simulink model "Wind_Harness"  (R2025b)
settings: Solver=VariableStepAuto  StartTime=0.0  StopTime=5  FixedStep=5e-5  RelTol=1e-3
PostLoadFcn:
  | WindFarmParam;
values from neighbouring files (symbols this model uses):
  base = struct    [WindFarmParam.m]
  pmsm = struct    [WindFarmParam.m]
  Ts = 5E-5    (= 5e-05)    [BESSGFLParam.m]    (also in BESSGFMParam.m; WindFarmParam.m)
  windController = struct    [WindFarmParam.m]
  windSystem = struct    [WindFarmParam.m]
  windTurbine = saveVarsMat.windTurbine    [WindFarmParam.m]
undefined symbols (not defined in the file or in its folder): DiscIntNeverNeededParam, Inertia
libraries: nesl_utility x34, fl_lib x18, ee_lib x18, eeTransforms x6, eeGeneralControl x5, simulink x4, eePwmGenerator x2, eeSinusoidalMeasurementV2 x1, eePmsmCurrentController x1, custom_lib x1
(part 2 of 2)

== system Wind_Harness/Wind Plant/Detailed/Wind Turbine and Converters/Wind Plant/Back-to-Back Converters ==
  Chopper : Inport
  SM_ref : Inport  Port=2
  Grid_ref : Inport  Port=3
  Average : Subsystem  VariantControl=Average
  Switching : Subsystem  VariantControl=Switching
  In : PMIOPort  Side=Left
  ~ : PMIOPort  Port=2  Side=Right
  Vdc : Outport

== system Wind_Harness/Wind Plant/Detailed/Wind Turbine and Converters/Wind Controller/Machine Converter Control/Measurements ==
  iabc_sens : Inport
  w_sens : Inport  Port=2
  th_sens : Inport  Port=3
  Vdc_sens : Inport  Port=4
  2*pi : Constant  Value=2*pi  SampleTime=-1
  Math Function : Math  Operator=mod  SignedPower=on
  pole pairs : Gain  Gain=p
  "pole pairs " : Gain  Gain=p
  we : Outport  VectorParamsAs1DForOutWhenUnconnected=off
  iabc : Outport  Port=2  VectorParamsAs1DForOutWhenUnconnected=off
  theta : Outport  Port=3  VectorParamsAs1DForOutWhenUnconnected=off
  Vdc : Outport  Port=4  VectorParamsAs1DForOutWhenUnconnected=off
  wires:
  Math Function/1 -> theta/1
  Vdc_sens/1 -> Vdc/1
  "pole pairs "/1 -> Math Function/1
  th_sens/1 -> "pole pairs "/1
  2*pi/1 -> Math Function/2
  pole pairs/1 -> we/1
  iabc_sens/1 -> iabc/1
  w_sens/1 -> pole pairs/1

== system Wind_Harness/Wind Plant/Detailed/Wind Turbine and Converters/Wind Controller/Machine Converter Control/Power Controller ==
  windSpeed : Inport
  Derating Control : Subsystem
  Greater than : simulink/Logic and Bit Operations/Compare To Constant  relop=>  const=12  OutDataTypeStr=boolean
  Less than or equal to : simulink/Logic and Bit Operations/Compare To Constant  relop=<=  const=12  OutDataTypeStr=boolean
  Limiter Function Power Demand : Subsystem
  MPPT Control : Subsystem
  activePowerDemand : Outport
  wires:
  Limiter Function Power Demand/1(activePowerDemand) -> activePowerDemand/1
  Derating Control/1(activePowerDemand) -> Limiter Function Power Demand/2(activePowerDemandDerating)
  MPPT Control/1(activePowerDemand) -> Limiter Function Power Demand/1(activePowerDemandMPPT)
  Greater than/1 -> Derating Control/Enable
  Less than or equal to/1 -> MPPT Control/Enable
  windSpeed/1 -> MPPT Control/1(windSpeed), Less than or equal to/1, Greater than/1

== system Wind_Harness/Wind Plant/Detailed/Wind Turbine and Converters/Wind Controller/Machine Converter Control/Subsystem ==
  note: LVRT Crowbar Control
  Vdc : Inport
  LVRT : Inport  Port=2
  Abs : Abs  SaturateOnIntegerOverflow=off
  Constant1 : Constant  Value=Vdc
  Product : Product
  Relay : Relay  OnSwitchValue=0.01001*Vdc  OffSwitchValue=0.01*Vdc
  Sum : Sum  Inputs=|+-
  Unit Delay1 : UnitDelay  SampleTime=-1  HasFrameUpgradeWarning=on
  Out1 : Outport
  wires:
  Relay/1 -> Out1/1
  Product/1 -> Abs/1
  LVRT/1 -> Product/2
  Unit Delay1/1 -> Sum/2
  Abs/1 -> Relay/1
  Sum/1 -> Product/1
  Vdc/1 -> Unit Delay1/1
  Constant1/1 -> Sum/1

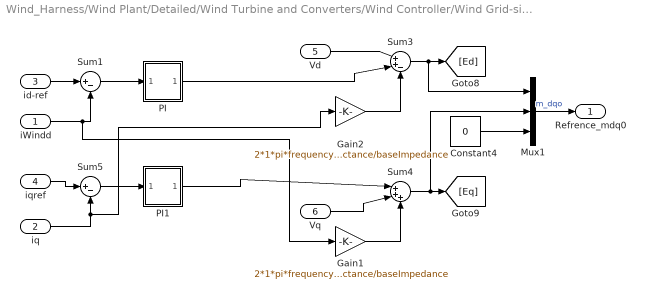
== system Wind_Harness/Wind Plant/Detailed/Wind Turbine and Converters/Wind Controller/Wind Grid-side Converter Controller/Current_controller ==
  iWindd : Inport
  iq : Inport  Port=2
  id-ref : Inport  Port=3
  iqref : Inport  Port=4
  Vd : Inport  Port=5
  Vq : Inport  Port=6
  Constant4 : Constant  Value=0
  Gain1 : Gain  Gain=2*1*pi*frequency*inductance/baseImpedance
  Gain2 : Gain  Gain=2*1*pi*frequency*inductance/baseImpedance
  Mux1 : Mux  Inputs=3
  PI : Subsystem
  PI1 : Subsystem
  Sum1 : Sum  Inputs=|+-
  Sum3 : Sum  Inputs=|++-
  Sum4 : Sum  Inputs=|+++
  Sum5 : Sum  Inputs=|+-
  Refrence_mdq0 : Outport
  wires:
  Mux1/1 -> Refrence_mdq0/1  "m_dqo"
  Sum4/1 -> [Eq], Mux1/2
  PI1/1(Out2) -> Sum4/1
  iqref/1 -> Sum5/1
  Sum5/1 -> PI1/1(Input)
  Constant4/1 -> Mux1/3
  Vd/1 -> Sum3/1
  Sum1/1 -> PI/1(Input)
  iq/1 -> Sum5/2, Gain2/1
  Vq/1 -> Sum4/2
  Gain1/1 -> Sum4/3
  id-ref/1 -> Sum1/1
  iWindd/1 -> Sum1/2, Gain1/1
  Gain2/1 -> Sum3/3
  Sum3/1 -> [Ed], Mux1/1
  PI/1(Out2) -> Sum3/2

== system Wind_Harness/Wind Plant/Detailed/Wind Turbine and Converters/Wind Controller/Wind Grid-side Converter Controller/DC Bus Chopper control  ==
  note: LVRT Detection
  In1 : Inport
  Constant1 : Constant
  Constant2 : Constant  Value=0
  Switch : Switch  Criteria=u2 > Threshold  Threshold=0.9  SaturateOnIntegerOverflow=off  InputSameDT=off
  Unit Delay : UnitDelay  SampleTime=-1  HasFrameUpgradeWarning=on
  Out1 : Outport
  wires:
  Unit Delay/1 -> Switch/2
  In1/1 -> Unit Delay/1
  Constant2/1 -> Switch/1
  Constant1/1 -> Switch/3
  Switch/1 -> Out1/1

== system Wind_Harness/Wind Plant/Detailed/Wind Turbine and Converters/Wind Controller/Wind Grid-side Converter Controller/DC voltage controller & current reference ==
  note: id_ref_generator
  note: iq_ref_generator
  note: Limiter
  Q_ref : Inport
  Vmag : Inport  Port=2
  Wind_Mpp_vdc : Inport  Port=3
  Wind_vdc : Inport  Port=4
  lvrt.iq : Inport  Port=5
  Constant : Constant
  Constant1 : Constant  Value=iMaxPU
  Current limits : Subsystem
  Subsystem : Subsystem
  Subsystem1 : Subsystem
  Switch : Switch  Criteria=u2 > Threshold  SaturateOnIntegerOverflow=off  InputSameDT=off
  Unit Delay1 : UnitDelay  SampleTime=Ts  HasFrameUpgradeWarning=on
  Unit Delay3 : UnitDelay  SampleTime=Ts  HasFrameUpgradeWarning=on
  id_ref : Outport
  iq_ref : Outport  Port=2
  wires:
  Constant/1 -> Switch/3
  Switch/1 -> Subsystem/1(V_mag)
  Vmag/1 -> Switch/2, Switch/1
  lvrt.iq/1 -> Subsystem/3(lvrt.iq)
  Current limits/1(iubq) -> Subsystem/2(iq_ub)
  Wind_vdc/1 -> Subsystem1/2(Wind_vdc)
  Wind_Mpp_vdc/1 -> Subsystem1/1(Wind_Mpp_vdc)
  Q_ref/1 -> Subsystem/4(Q_ref)
  Unit Delay3/1 -> Current limits/3(idref)
  Subsystem1/1(Out1) -> Unit Delay3/1, id_ref/1
  Unit Delay1/1 -> Current limits/2(iqref)
  Constant1/1 -> Current limits/1(Imax)
  Subsystem/1(Out1) -> iq_ref/1, Unit Delay1/1
  Current limits/2(iubd) -> Subsystem1/3(id_ub)

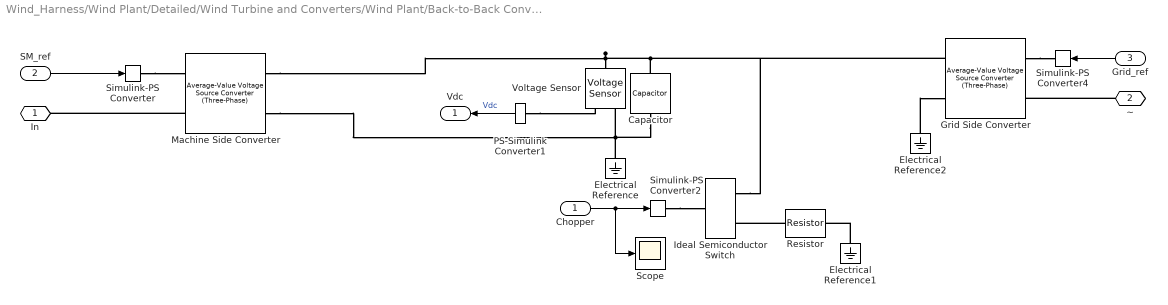
== system Wind_Harness/Wind Plant/Detailed/Wind Turbine and Converters/Wind Plant/Back-to-Back Converters/Average ==
  Chopper : Inport
  SM_ref : Inport  Port=2
  Grid_ref : Inport  Port=3
  Capacitor : fl_lib/Electrical/Electrical Elements/Capacitor  c=capDC F  r=1e-1 Ohm  g=0 1/Ohm  i_specify=off  i_priority=None  i=0 A  i_nominal_specify=off  i_nominal_value=1  i_nominal_unit=A  v_specify=off  v_priority=None  v=0 V  v_nominal_specify=off  v_nominal_value=1  v_nominal_unit=V  vc_specify=on  vc_priority=High  vc=Vdc V  vc_nominal_specify=off  vc_nominal_value=1  vc_nominal_unit=V
  Electrical Reference : fl_lib/Electrical/Electrical Elements/Electrical Reference
  Electrical Reference1 : fl_lib/Electrical/Electrical Elements/Electrical Reference
  Electrical Reference2 : fl_lib/Electrical/Electrical Elements/Electrical Reference
  Grid Side Converter : ee_lib/Semiconductors & Converters/Converters/Average-Value Voltage Source Converter (Three-Phase)  port_option=ee.enum.threePhasePort.composite  frequency_option=ee.enum.converters.frequency.variable  input_option=ee.enum.converters.inputOption.ModWave  FRated=60 Hz  losses_parameterization=ee.enum.converters.losses.fixed  Pfixed=1 W  ks=0.01  kc1=1.7 V  kc2=0.01 Ohm  Ploss_vect=[100, 800, 1870, 3250, 4900] W  Irms_vect=[10, 100, 200, 300, 400] A  Vdc_nom=300 V  thermal_mass=30000 J/K  temperature_specify=off  temperature_priority=High  temperature=298.15 K  temperature_nominal_specify=off  temperature_nominal_value=1  temperature_nominal_unit=K
      settings: InternalSimscapePortConfiguration="{\"Bottom\":[],\"Left\":[{\"id\":\"ModWave\",\"label\":\"ModWave\",\"type\":\"input\"},{\"id\":\"N\",\"label\":\"~\",\"type\":\"foundation.electrical.three_phase\"}],\"Right\":[{\"id\":\"p\",\"label\":\"+\",\"type\":\"foundation.electrical.electrical\"},{\"id\":\"n\",\"label\":\"-\",\"type\":\"foundation.electrical.electrical\"}],\"Top\":[]}"
  Ideal Semiconductor Switch : ee_lib/Semiconductors & Converters/Ideal Semiconductor Switch  port_option=ee.enum.controlport.ps  Ron=0.001 Ohm  Goff=1e-6 1/Ohm  Vth=0.5 V  diode_param=ee.enum.converters.protectiondiode.none  diode_Vf=0.8 V  diode_Ron=0.001 Ohm  diode_Goff=1e-5 1/Ohm  diode_C=50e-9 F  diode_iRM=-235 A  diode_iF=300 A  diode_idot=-50 A/us  diode_trr_param=ee.enum.converters.diodetrr.trr_factor  diode_trr_factor=3  diode_trr=15 us  diode_Qrr=1500 s*uA
  Machine Side Converter : ee_lib/Semiconductors & Converters/Converters/Average-Value Voltage Source Converter (Three-Phase)  port_option=ee.enum.threePhasePort.composite  frequency_option=ee.enum.converters.frequency.variable  input_option=ee.enum.converters.inputOption.ModWave  FRated=60 Hz  losses_parameterization=ee.enum.converters.losses.fixed  Pfixed=1 W  ks=0.01  kc1=1.7 V  kc2=0.01 Ohm  Ploss_vect=[100, 800, 1870, 3250, 4900] W  Irms_vect=[10, 100, 200, 300, 400] A  Vdc_nom=300 V  thermal_mass=30000 J/K  temperature_specify=off  temperature_priority=High  temperature=298.15 K  temperature_nominal_specify=off  temperature_nominal_value=1  temperature_nominal_unit=K
      settings: InternalSimscapePortConfiguration="{\"Bottom\":[],\"Left\":[{\"id\":\"ModWave\",\"label\":\"ModWave\",\"type\":\"input\"},{\"id\":\"N\",\"label\":\"~\",\"type\":\"foundation.electrical.three_phase\"}],\"Right\":[{\"id\":\"p\",\"label\":\"+\",\"type\":\"foundation.electrical.electrical\"},{\"id\":\"n\",\"label\":\"-\",\"type\":\"foundation.electrical.electrical\"}],\"Top\":[]}"
  PS-Simulink Converter1 : nesl_utility/PS-Simulink Converter  PhysicalDomain=network_engine_domain  SubClassName=ps_output  LeftPortType=input  RightPortType=output  PseudoPeriodic=off  Frequencies=[]  VectorFormat=1-D array  Unit=V  AffineConversion=off
  Resistor : fl_lib/Electrical/Electrical Elements/Resistor  R=16 Ohm  i_specify=off  i_priority=None  i=0 A  i_nominal_specify=off  i_nominal_value=1  i_nominal_unit=A  v_specify=off  v_priority=None  v=0 V  v_nominal_specify=off  v_nominal_value=1  v_nominal_unit=V
  Scope : Scope
      settings: ActiveDisplayYMinimum=-0.125  ActiveDisplayYMaximum=1.125  DataLoggingVariableName=ScopeData11
  Simulink-PS Converter : nesl_utility/Simulink-PS Converter  PhysicalDomain=network_engine_domain  SubClassName=ps_input  LeftPortType=input  RightPortType=output  PseudoPeriodic=off  Frequencies=[]  NoiseDistribution=none  NoiseParameters=[]  Unit=1  AffineConversion=off  FilteringAndDerivatives=provide  SimscapeFilterOrder=1  InputFilterTimeConstant=0.001  UdotUserProvided=0
  Simulink-PS Converter2 : nesl_utility/Simulink-PS Converter  PhysicalDomain=network_engine_domain  SubClassName=ps_input  LeftPortType=input  RightPortType=output  PseudoPeriodic=off  Frequencies=[]  NoiseDistribution=none  NoiseParameters=[]  Unit=1  AffineConversion=off  FilteringAndDerivatives=provide  SimscapeFilterOrder=1  InputFilterTimeConstant=0.001  UdotUserProvided=0
  Simulink-PS Converter4 : nesl_utility/Simulink-PS Converter  PhysicalDomain=network_engine_domain  SubClassName=ps_input  LeftPortType=input  RightPortType=output  PseudoPeriodic=off  Frequencies=[]  NoiseDistribution=none  NoiseParameters=[]  Unit=1  AffineConversion=off  FilteringAndDerivatives=provide  SimscapeFilterOrder=1  InputFilterTimeConstant=0.001  UdotUserProvided=0
  Voltage Sensor : fl_lib/Electrical/Electrical Sensors/Voltage Sensor
  In : PMIOPort  Side=Left
  ~ : PMIOPort  Port=2  Side=Right
  Vdc : Outport
  wires:
  SM_ref/1 -> Simulink-PS Converter/1
  PS-Simulink Converter1/1 -> Vdc/1  "Vdc"
  Chopper/1 -> Simulink-PS Converter2/1, Scope/1
  Grid_ref/1 -> Simulink-PS Converter4/1
  connections:
  Simulink-PS Converter/RConn1 -- Machine Side Converter/LConn1
  Machine Side Converter/LConn2 -- In/RConn1
  Simulink-PS Converter2/RConn1 -- Ideal Semiconductor Switch/LConn1
  Electrical Reference1/LConn1 -- Resistor/RConn1
  Grid Side Converter/LConn1 -- Simulink-PS Converter4/RConn1
  Resistor/LConn1 -- Ideal Semiconductor Switch/RConn2
  ~/RConn1 -- Grid Side Converter/LConn2
  PS-Simulink Converter1/LConn1 -- Voltage Sensor/RConn1
  Electrical Reference2/LConn1 -- Grid Side Converter/RConn2
  Voltage Sensor/LConn1 -- Machine Side Converter/RConn1 -- Ideal Semiconductor Switch/RConn1 -- Grid Side Converter/RConn1 -- Capacitor/LConn1
  Capacitor/RConn1 -- Voltage Sensor/RConn2 -- Machine Side Converter/RConn2 -- Electrical Reference/LConn1

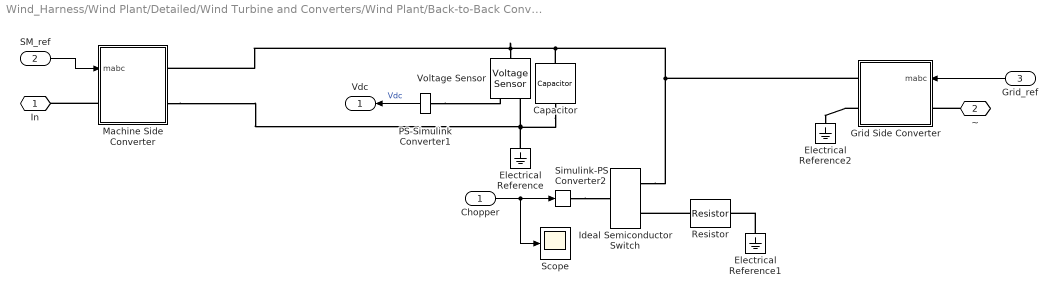
== system Wind_Harness/Wind Plant/Detailed/Wind Turbine and Converters/Wind Plant/Back-to-Back Converters/Switching ==
  Chopper : Inport
  SM_ref : Inport  Port=2
  Grid_ref : Inport  Port=3
  Capacitor : fl_lib/Electrical/Electrical Elements/Capacitor  c=capacitance F  r=1e-1 Ohm  g=0 1/Ohm  i_specify=off  i_priority=None  i=0 A  i_nominal_specify=off  i_nominal_value=1  i_nominal_unit=A  v_specify=off  v_priority=None  v=0 V  v_nominal_specify=off  v_nominal_value=1  v_nominal_unit=V  vc_specify=on  vc_priority=High  vc=baseVoltageDC V  vc_nominal_specify=off  vc_nominal_value=1  vc_nominal_unit=V
  Electrical Reference : fl_lib/Electrical/Electrical Elements/Electrical Reference
  Electrical Reference1 : fl_lib/Electrical/Electrical Elements/Electrical Reference
  Electrical Reference2 : fl_lib/Electrical/Electrical Elements/Electrical Reference
  Grid Side Converter : Subsystem
      settings: PortSchema="{\"entries\":[{\"content\":{\"sides\":[{\"content\":{\"connectorIds\":[\"LConn1\",\"LConn2\"]},\"type\":\"ConnectorPlacement.EquallySpacedRectSide\",\"uuid\":\"e32be008-cebd-46aa-ba62-c5c92b9b23e3\"},{\"content\":{\"connectorIds\":[\"In1\",\"RConn1\"],\"side\":\"RIGHT\"},\"type\":\"ConnectorPlacement.EquallySpacedRectSide\",\"uuid\":\"c483e451-04b5-4212-bdd1-c589ba5bea78\"},{\"content\":{\"side\":\"TOP\"},\"type\":\"ConnectorPlacement.EquallySpacedRectSide\",\"uuid\":\"824c135c-7e5f-4da0-a7de-e626b4bfa50d\"}]},\"type\":\"ConnectorPlacement.EquallySpacedConnector\",\"uuid\":\"5f81c72d-92ab-4525-91a6-193f769a7c86\"}],\"packageUris\":[\"http://schema.mathworks.com/mf0/Connector/R2020b\"],\"version\":\"1.0\"}"
  Ideal Semiconductor Switch : ee_lib/Semiconductors & Converters/Ideal Semiconductor Switch  port_option=ee.enum.controlport.ps  Ron=0.001 Ohm  Goff=1e-6 1/Ohm  Vth=0.5 V  diode_param=ee.enum.converters.protectiondiode.none  diode_Vf=0.8 V  diode_Ron=0.001 Ohm  diode_Goff=1e-5 1/Ohm  diode_C=50e-9 F  diode_iRM=-235 A  diode_iF=300 A  diode_idot=-50 A/us  diode_trr_param=ee.enum.converters.diodetrr.trr_factor  diode_trr_factor=3  diode_trr=15 us  diode_Qrr=1500 s*uA
  Machine Side Converter : Subsystem
      settings: PortSchema="{\"entries\":[{\"content\":{\"sides\":[{\"content\":{\"connectorIds\":[\"LConn1\",\"LConn2\"]},\"type\":\"ConnectorPlacement.EquallySpacedRectSide\",\"uuid\":\"e32be008-cebd-46aa-ba62-c5c92b9b23e3\"},{\"content\":{\"connectorIds\":[\"In1\",\"RConn1\"],\"side\":\"RIGHT\"},\"type\":\"ConnectorPlacement.EquallySpacedRectSide\",\"uuid\":\"c483e451-04b5-4212-bdd1-c589ba5bea78\"},{\"content\":{\"side\":\"TOP\"},\"type\":\"ConnectorPlacement.EquallySpacedRectSide\",\"uuid\":\"824c135c-7e5f-4da0-a7de-e626b4bfa50d\"}]},\"type\":\"ConnectorPlacement.EquallySpacedConnector\",\"uuid\":\"5f81c72d-92ab-4525-91a6-193f769a7c86\"}],\"packageUris\":[\"http://schema.mathworks.com/mf0/Connector/R2020b\"],\"version\":\"1.0\"}"
  PS-Simulink Converter1 : nesl_utility/PS-Simulink Converter  PhysicalDomain=network_engine_domain  SubClassName=ps_output  LeftPortType=input  RightPortType=output  PseudoPeriodic=off  Frequencies=[]  VectorFormat=1-D array  Unit=V  AffineConversion=off
  Resistor : fl_lib/Electrical/Electrical Elements/Resistor  R=16 Ohm  i_specify=off  i_priority=None  i=0 A  i_nominal_specify=off  i_nominal_value=1  i_nominal_unit=A  v_specify=off  v_priority=None  v=0 V  v_nominal_specify=off  v_nominal_value=1  v_nominal_unit=V
  Scope : Scope
      settings: ActiveDisplayYMinimum=-0.125  ActiveDisplayYMaximum=1.125  DataLoggingVariableName=ScopeData11
  Simulink-PS Converter2 : nesl_utility/Simulink-PS Converter  PhysicalDomain=network_engine_domain  SubClassName=ps_input  LeftPortType=input  RightPortType=output  PseudoPeriodic=off  Frequencies=[]  NoiseDistribution=none  NoiseParameters=[]  Unit=1  AffineConversion=off  FilteringAndDerivatives=provide  SimscapeFilterOrder=1  InputFilterTimeConstant=0.001  UdotUserProvided=0
  Voltage Sensor : fl_lib/Electrical/Electrical Sensors/Voltage Sensor
  In : PMIOPort  Side=Left
  ~ : PMIOPort  Port=2  Side=Right
  Vdc : Outport
  wires:
  PS-Simulink Converter1/1 -> Vdc/1  "Vdc"
  Chopper/1 -> Simulink-PS Converter2/1, Scope/1
  Grid_ref/1 -> Grid Side Converter/1(mabc)
  SM_ref/1 -> Machine Side Converter/1(mabc)
  connections:
  Machine Side Converter/RConn1 -- In/RConn1
  Simulink-PS Converter2/RConn1 -- Ideal Semiconductor Switch/LConn1
  Electrical Reference1/LConn1 -- Resistor/RConn1
  Resistor/LConn1 -- Ideal Semiconductor Switch/RConn2
  ~/RConn1 -- Grid Side Converter/RConn1
  PS-Simulink Converter1/LConn1 -- Voltage Sensor/RConn1
  Grid Side Converter/LConn2 -- Electrical Reference2/LConn1
  Voltage Sensor/LConn1 -- Machine Side Converter/LConn1 -- Capacitor/LConn1 -- Grid Side Converter/LConn1 -- Ideal Semiconductor Switch/RConn1
  Electrical Reference/LConn1 -- Voltage Sensor/RConn2 -- Machine Side Converter/LConn2 -- Capacitor/RConn1

== system Wind_Harness/Wind Plant/Detailed/Wind Turbine and Converters/Wind Controller/Machine Converter Control/Power Controller/Derating Control ==
  Enable : EnablePort  StatesWhenEnabling=reset
  Constant : Constant  Value=windTurbine.turbineRatedPower
  MW to W : Gain  Gain=1e6
  activePowerDemand : Outport
  wires:
  Constant/1 -> MW to W/1
  MW to W/1 -> activePowerDemand/1

== system Wind_Harness/Wind Plant/Detailed/Wind Turbine and Converters/Wind Controller/Machine Converter Control/Power Controller/Limiter Function Power Demand ==
  activePowerDemandMPPT : Inport
  activePowerDemandDerating : Inport  Port=2
  Merge : Merge
  activePowerDemand : Outport
  wires:
  Merge/1 -> activePowerDemand/1
  activePowerDemandDerating/1 -> Merge/2
  activePowerDemandMPPT/1 -> Merge/1

== system Wind_Harness/Wind Plant/Detailed/Wind Turbine and Converters/Wind Controller/Machine Converter Control/Power Controller/MPPT Control ==
  windSpeed : Inport
  Enable : EnablePort  StatesWhenEnabling=reset
  MW to W : Gain  Gain=1e6
  mpptActivePowerDemand : Lookup_n-D  NumberOfTableDimensions=1  BreakpointsForDimension1=mpptWindSpeed  Table=mpptPower  InternalRulePriority=Speed  RndMeth=Simplest
  activePowerDemand : Outport
  wires:
  MW to W/1 -> activePowerDemand/1
  windSpeed/1 -> mpptActivePowerDemand/1
  mpptActivePowerDemand/1 -> MW to W/1

== system Wind_Harness/Wind Plant/Detailed/Wind Turbine and Converters/Wind Controller/Wind Grid-side Converter Controller/Current_controller/PI ==
  Input : Inport
  Discrete-Time Integrator : DiscreteIntegrator  gainval=Kdii_g  SampleTime=Ts  ICPrevOutput=DiscIntNeverNeededParam  ICPrevScaledInput=DiscIntNeverNeededParam
  Gain1 : Gain  Gain=Kdpi_g
  Sum1 : Sum  Inputs=|++
  Unit Delay : UnitDelay  SampleTime=Ts  HasFrameUpgradeWarning=on
  Out2 : Outport
  wires:
  Input/1 -> Discrete-Time Integrator/1, Gain1/1
  Gain1/1 -> Unit Delay/1
  Unit Delay/1 -> Sum1/2
  Sum1/1 -> Out2/1
  Discrete-Time Integrator/1 -> Sum1/1

== system Wind_Harness/Wind Plant/Detailed/Wind Turbine and Converters/Wind Controller/Wind Grid-side Converter Controller/Current_controller/PI1 ==
  Input : Inport
  Discrete-Time Integrator : DiscreteIntegrator  gainval=Kqii_g  SampleTime=Ts  ICPrevOutput=DiscIntNeverNeededParam  ICPrevScaledInput=DiscIntNeverNeededParam
  Gain1 : Gain  Gain=Kqpi_g
  Sum1 : Sum  Inputs=|++
  Unit Delay : UnitDelay  SampleTime=Ts  HasFrameUpgradeWarning=on
  Out2 : Outport
  wires:
  Input/1 -> Discrete-Time Integrator/1, Gain1/1
  Gain1/1 -> Unit Delay/1
  Unit Delay/1 -> Sum1/2
  Sum1/1 -> Out2/1
  Discrete-Time Integrator/1 -> Sum1/1

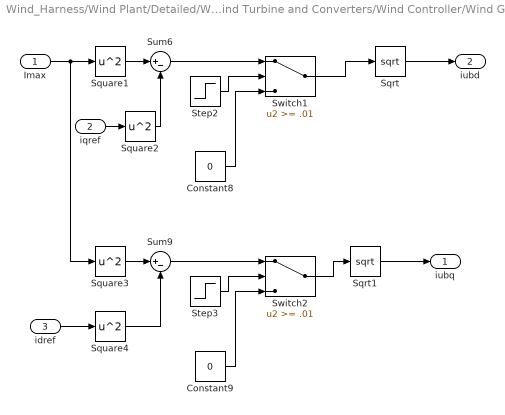
== system Wind_Harness/Wind Plant/Detailed/Wind Turbine and Converters/Wind Controller/Wind Grid-side Converter Controller/DC voltage controller & current reference/Current limits ==
  Imax : Inport
  iqref : Inport  Port=2
  idref : Inport  Port=3
  Constant8 : Constant  Value=0
  Constant9 : Constant  Value=0
  Sqrt : Sqrt
  Sqrt1 : Sqrt
  Square{1..4} (4 alike) : Math  Operator=square
  Step2 : Step  Time=0.01  SampleTime=Ts
  Step3 : Step  Time=0.01  SampleTime=Ts
  Sum6 : Sum  Inputs=|+-
  Sum9 : Sum  Inputs=|+-
  Switch1 : Switch  Threshold=.01  SaturateOnIntegerOverflow=off  InputSameDT=off
  Switch2 : Switch  Threshold=.01  SaturateOnIntegerOverflow=off  InputSameDT=off
  iubq : Outport
  iubd : Outport  Port=2
  wires:
  idref/1 -> Square4/1
  Sqrt1/1 -> iubq/1
  Imax/1 -> Square1/1, Square3/1
  Sqrt/1 -> iubd/1
  Constant9/1 -> Switch2/3
  Square4/1 -> Sum9/2
  Constant8/1 -> Switch1/3
  Square2/1 -> Sum6/2
  Sum6/1 -> Switch1/1
  Square3/1 -> Sum9/1
  iqref/1 -> Square2/1
  Switch1/1 -> Sqrt/1
  Square1/1 -> Sum6/1
  Switch2/1 -> Sqrt1/1
  Step2/1 -> Switch1/2
  Step3/1 -> Switch2/2
  Sum9/1 -> Switch2/1

== system Wind_Harness/Wind Plant/Detailed/Wind Turbine and Converters/Wind Controller/Wind Grid-side Converter Controller/DC voltage controller & current reference/Subsystem ==
  V_mag : Inport
  iq_ub : Inport  Port=2
  lvrt.iq : Inport  Port=3
  Q_ref : Inport  Port=4
  Divide2 : Product  Inputs=*/
  Gain3 : Gain  Gain=-1
  Saturation Dynamic2 : simulink/Discontinuities/Saturation Dynamic  OutMin=[]  OutMax=[]  OutDataTypeStr=Inherit: Same as second input  OutDataType=fixdt(1, 16)  OutScaling=2^-10  DoSatur=off
  Switch6 : Switch  Threshold=.9  SaturateOnIntegerOverflow=off  InputSameDT=off
  iq_ub1 : InportShadow  Port=2
  Out1 : Outport
  wires:
  lvrt.iq/1 -> Switch6/3
  Switch6/1 -> Out1/1
  Saturation Dynamic2/1 -> Switch6/1
  iq_ub/1 -> Saturation Dynamic2/1
  Gain3/1 -> Saturation Dynamic2/3
  Q_ref/1 -> Divide2/1
  Divide2/1 -> Saturation Dynamic2/2
  iq_ub1/1 -> Gain3/1
  V_mag/1 -> Divide2/2, Switch6/2

== system Wind_Harness/Wind Plant/Detailed/Wind Turbine and Converters/Wind Controller/Wind Grid-side Converter Controller/DC voltage controller & current reference/Subsystem1 ==
  Wind_Mpp_vdc : Inport
  Wind_vdc : Inport  Port=2
  id_ub : Inport  Port=3
  Constant4 : Constant  Value=0
  Saturation Dynamic1 : simulink/Discontinuities/Saturation Dynamic  OutMin=[]  OutMax=[]  OutDataTypeStr=Inherit: Same as second input  OutDataType=fixdt(1, 16)  OutScaling=2^-10  DoSatur=off
  V_dc_Controller1 : Subsystem
  Out1 : Outport
  wires:
  Wind_Mpp_vdc/1 -> V_dc_Controller1/1(Wind_plant1)
  Saturation Dynamic1/1 -> Out1/1
  id_ub/1 -> Saturation Dynamic1/1
  Wind_vdc/1 -> V_dc_Controller1/2(In2)
  V_dc_Controller1/1(Out1) -> Saturation Dynamic1/2
  Constant4/1 -> Saturation Dynamic1/3

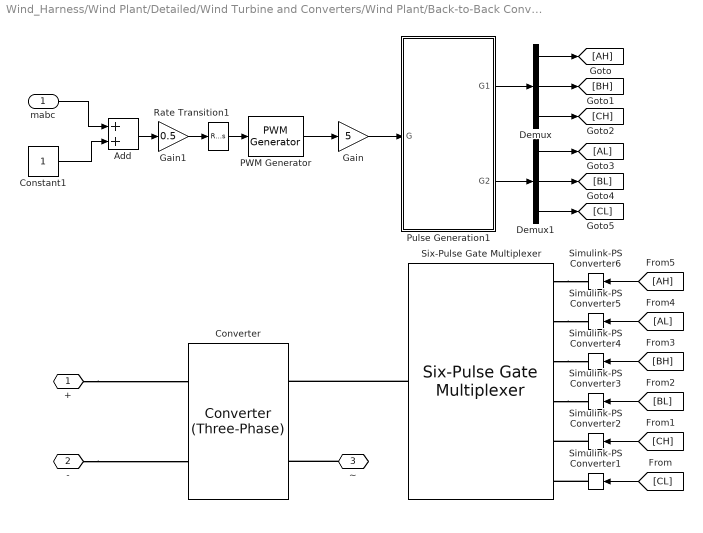
== system Wind_Harness/Wind Plant/Detailed/Wind Turbine and Converters/Wind Plant/Back-to-Back Converters/Switching/Grid Side Converter ==
  mabc : Inport
  Add : Sum
  Constant1 : Constant
  Converter : ee_lib/Semiconductors & Converters/Converters/Converter (Three-Phase)  port_option=ee.enum.threePhasePort.composite  fidelity_option=ee.enum.converters.fidelity.detailed  device_type=ee.enum.converters.switchingdevice.ideal  showThermalPort=false  K=0  Vth=1 V  Vgt=1 V  Vgt_off=-1 V  Ih=1 A  Vf=0.8 V  Ron=0.001 Ohm  Rds=0.001 Ohm  Goff=1e-6 1/Ohm  Eon_scalar=22.86e-3 J  Eoff_scalar=17.14e-3 J  Eoff_natural_commutation=10e-3 J  Voff=300 V  Iout_scalar=600 A  onCurrentMeasDelay=0 s  useCurrentFromPreviousCycle=false  useVoltageFromPreviousCycle=false  diode_param=ee.enum.converters.protectiondiode.nodynamics  diode_Vf=0.01 V  diode_Ron=0.0001 Ohm  diode_Goff=1e-5 1/Ohm  diode_C=50 nF  diode_iRM=-235 A  diode_iF=300 A  diode_idot=-50 A/us  diode_trr_param=ee.enum.converters.diodetrr.trr_factor  diode_trr_factor=3  diode_trr=15 us  diode_Qrr=1500 s*uA  diode_rec_loss_model=ee.enum.diode.reverseRecoveryModel.fixed  diode_ErecVal=0 J  diode_scaleWithIandV=false  diode_ErecMat=zeros(2, 3) J  diode_TjrecVec=[298.15, 398.15] K  diode_IfrecVec=[.1, 1, 10] A  diode_IrecVal=10 A  diode_VrecVal=10 V  diode_tFilter=1 / 1000 / 100 s  thermal_network_parameterization=ee.enum.thermalNetworkTopology.external  Rth=[.08, .5] K/W  Rth_Cauer=[.08, .1, .5] K/W  Rth_Foster=[.08, .14, .22, .16] K/W  thermal_mass_parameterization=ee.enum.thermalNetwork.timeconstant  thermal_mass=[.01, .5] J/K  thermal_mass_Cauer=[.01, .1, .5] J/K  thermal_mass_Foster=[.001, .005, .05, .5] J/K  thermal_time_constant=[.001, .2] s  thermal_time_constant_Cauer=[.001, .1, .2] s  thermal_time_constant_Foster=[7e-05, .0007, .01, .08] s  thermal_mass_initial_temperatures=[25, 25] degC  thermal_mass_initial_temperatures_Cauer=[25, 25, 25] degC  junction_thermal_mass=0.01 J/K  Tvec_initial_Foster=[25, 25, 25, 25] degC  snubber_type=ee.enum.converters.snubber.exclude  Cs=1e-7 F  Rs=0.1 Ohm  Vce_loss=[0, 150, 300] V
  Demux : Demux  Outputs=3
  Demux1 : Demux  Outputs=3
  Gain : Gain  Gain=5
  Gain1 : Gain  Gain=0.5
  PWM Generator : eePwmGenerator/PWM Generator  CarrCount=Up  Tper=1/(fSw*1000)  Tdelay=0  Ts=1/(10*fSw*1000)
  Pulse Generation1 : Subsystem
  Rate Transition1 : RateTransition  OutPortSampleTime=1/(10*fSw*1000)
  Simulink-PS Converter{1..6} (6 alike) : nesl_utility/Simulink-PS Converter  PhysicalDomain=network_engine_domain  SubClassName=ps_input  LeftPortType=input  RightPortType=output  PseudoPeriodic=off  Frequencies=[]  NoiseDistribution=none  NoiseParameters=[]  Unit=1  AffineConversion=off  FilteringAndDerivatives=provide  SimscapeFilterOrder=1  InputFilterTimeConstant=0.001  UdotUserProvided=0
  Six-Pulse Gate Multiplexer : ee_lib/Semiconductors & Converters/Converters/Six-Pulse Gate Multiplexer  port_option=ee.enum.controlport.ps
  + : PMIOPort  Side=Left
  - : PMIOPort  Port=2  Side=Left
  ~ : PMIOPort  Port=3  Side=Right
  wires:
  [CH] -> Simulink-PS Converter2/1
  Demux/1 -> [AH]
  Add/1 -> Gain1/1
  Constant1/1 -> Add/2
  Demux/3 -> [CH]
  [AH] -> Simulink-PS Converter6/1
  Rate Transition1/1 -> PWM Generator/1
  [BH] -> Simulink-PS Converter4/1
  Demux1/3 -> [CL]
  [CL] -> Simulink-PS Converter1/1
  [AL] -> Simulink-PS Converter5/1
  PWM Generator/1 -> Gain/1
  Gain1/1 -> Rate Transition1/1
  Demux1/2 -> [BL]
  Demux/2 -> [BH]
  mabc/1 -> Add/1
  Gain/1 -> Pulse Generation1/1(G)
  Demux1/1 -> [AL]
  Pulse Generation1/2(G2) -> Demux1/1
  Pulse Generation1/1(G1) -> Demux/1
  [BL] -> Simulink-PS Converter3/1
  connections:
  +/RConn1 -- Converter/RConn1
  Six-Pulse Gate Multiplexer/LConn1 -- Simulink-PS Converter6/RConn1
  -/RConn1 -- Converter/RConn2
  Simulink-PS Converter2/RConn1 -- Six-Pulse Gate Multiplexer/LConn5
  Six-Pulse Gate Multiplexer/LConn3 -- Simulink-PS Converter4/RConn1
  Six-Pulse Gate Multiplexer/LConn2 -- Simulink-PS Converter5/RConn1
  Six-Pulse Gate Multiplexer/RConn1 -- Converter/LConn1
  ~/RConn1 -- Converter/LConn2
  Six-Pulse Gate Multiplexer/LConn4 -- Simulink-PS Converter3/RConn1
  Simulink-PS Converter1/RConn1 -- Six-Pulse Gate Multiplexer/LConn6

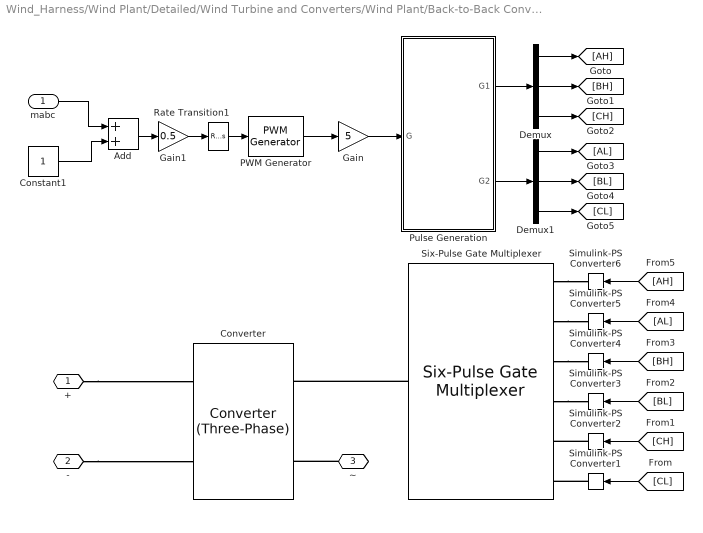
== system Wind_Harness/Wind Plant/Detailed/Wind Turbine and Converters/Wind Plant/Back-to-Back Converters/Switching/Machine Side Converter ==
  mabc : Inport
  Add : Sum
  Constant1 : Constant
  Converter : ee_lib/Semiconductors & Converters/Converters/Converter (Three-Phase)  port_option=ee.enum.threePhasePort.composite  fidelity_option=ee.enum.converters.fidelity.detailed  device_type=ee.enum.converters.switchingdevice.ideal  showThermalPort=false  K=0  Vth=1 V  Vgt=1 V  Vgt_off=-1 V  Ih=1 A  Vf=0.8 V  Ron=0.001 Ohm  Rds=0.001 Ohm  Goff=1e-6 1/Ohm  Eon_scalar=22.86e-3 J  Eoff_scalar=17.14e-3 J  Eoff_natural_commutation=10e-3 J  Voff=300 V  Iout_scalar=600 A  onCurrentMeasDelay=0 s  useCurrentFromPreviousCycle=false  useVoltageFromPreviousCycle=false  diode_param=ee.enum.converters.protectiondiode.nodynamics  diode_Vf=0.01 V  diode_Ron=0.0001 Ohm  diode_Goff=1e-5 1/Ohm  diode_C=50 nF  diode_iRM=-235 A  diode_iF=300 A  diode_idot=-50 A/us  diode_trr_param=ee.enum.converters.diodetrr.trr_factor  diode_trr_factor=3  diode_trr=15 us  diode_Qrr=1500 s*uA  diode_rec_loss_model=ee.enum.diode.reverseRecoveryModel.fixed  diode_ErecVal=0 J  diode_scaleWithIandV=false  diode_ErecMat=zeros(2, 3) J  diode_TjrecVec=[298.15, 398.15] K  diode_IfrecVec=[.1, 1, 10] A  diode_IrecVal=10 A  diode_VrecVal=10 V  diode_tFilter=1 / 1000 / 100 s  thermal_network_parameterization=ee.enum.thermalNetworkTopology.external  Rth=[.08, .5] K/W  Rth_Cauer=[.08, .1, .5] K/W  Rth_Foster=[.08, .14, .22, .16] K/W  thermal_mass_parameterization=ee.enum.thermalNetwork.timeconstant  thermal_mass=[.01, .5] J/K  thermal_mass_Cauer=[.01, .1, .5] J/K  thermal_mass_Foster=[.001, .005, .05, .5] J/K  thermal_time_constant=[.001, .2] s  thermal_time_constant_Cauer=[.001, .1, .2] s  thermal_time_constant_Foster=[7e-05, .0007, .01, .08] s  thermal_mass_initial_temperatures=[25, 25] degC  thermal_mass_initial_temperatures_Cauer=[25, 25, 25] degC  junction_thermal_mass=0.01 J/K  Tvec_initial_Foster=[25, 25, 25, 25] degC  snubber_type=ee.enum.converters.snubber.exclude  Cs=1e-7 F  Rs=0.1 Ohm  Vce_loss=[0, 150, 300] V
  Demux : Demux  Outputs=3
  Demux1 : Demux  Outputs=3
  Gain : Gain  Gain=5
  Gain1 : Gain  Gain=0.5
  PWM Generator : eePwmGenerator/PWM Generator  CarrCount=Up  Tper=1/(fSw*1000)  Tdelay=0  Ts=1/(10*fSw*1000)
  Pulse Generation : Subsystem
  Rate Transition1 : RateTransition  OutPortSampleTime=1/(10*fSw*1000)
  Simulink-PS Converter{1..6} (6 alike) : nesl_utility/Simulink-PS Converter  PhysicalDomain=network_engine_domain  SubClassName=ps_input  LeftPortType=input  RightPortType=output  PseudoPeriodic=off  Frequencies=[]  NoiseDistribution=none  NoiseParameters=[]  Unit=1  AffineConversion=off  FilteringAndDerivatives=provide  SimscapeFilterOrder=1  InputFilterTimeConstant=0.001  UdotUserProvided=0
  Six-Pulse Gate Multiplexer : ee_lib/Semiconductors & Converters/Converters/Six-Pulse Gate Multiplexer  port_option=ee.enum.controlport.ps
  + : PMIOPort  Side=Left
  - : PMIOPort  Port=2  Side=Left
  ~ : PMIOPort  Port=3  Side=Right
  wires:
  Demux1/1 -> [AL]
  Rate Transition1/1 -> PWM Generator/1
  Gain/1 -> Pulse Generation/1(G)
  [BH] -> Simulink-PS Converter4/1
  Gain1/1 -> Rate Transition1/1
  Demux/2 -> [BH]
  Pulse Generation/1(G1) -> Demux/1
  Pulse Generation/2(G2) -> Demux1/1
  PWM Generator/1 -> Gain/1
  Constant1/1 -> Add/2
  [AL] -> Simulink-PS Converter5/1
  Demux/3 -> [CH]
  [BL] -> Simulink-PS Converter3/1
  Demux/1 -> [AH]
  Add/1 -> Gain1/1
  Demux1/2 -> [BL]
  [CH] -> Simulink-PS Converter2/1
  Demux1/3 -> [CL]
  [CL] -> Simulink-PS Converter1/1
  mabc/1 -> Add/1
  [AH] -> Simulink-PS Converter6/1
  connections:
  Simulink-PS Converter2/RConn1 -- Six-Pulse Gate Multiplexer/LConn5
  ~/RConn1 -- Converter/LConn2
  Six-Pulse Gate Multiplexer/RConn1 -- Converter/LConn1
  Six-Pulse Gate Multiplexer/LConn2 -- Simulink-PS Converter5/RConn1
  Six-Pulse Gate Multiplexer/LConn4 -- Simulink-PS Converter3/RConn1
  -/RConn1 -- Converter/RConn2
  Six-Pulse Gate Multiplexer/LConn1 -- Simulink-PS Converter6/RConn1
  +/RConn1 -- Converter/RConn1
  Simulink-PS Converter1/RConn1 -- Six-Pulse Gate Multiplexer/LConn6
  Six-Pulse Gate Multiplexer/LConn3 -- Simulink-PS Converter4/RConn1

== system Wind_Harness/Wind Plant/Detailed/Wind Turbine and Converters/Wind Controller/Wind Grid-side Converter Controller/DC voltage controller & current reference/Subsystem1/V_dc_Controller1 ==
  Wind_plant1 : Inport
  In2 : Inport  Port=2
  Gain : Gain  Gain=1/Vdc
  PI : Subsystem
  Sum : Sum  Inputs=|+-
  Out1 : Outport
  wires:
  PI/1(Out2) -> Out1/1
  Gain/1 -> PI/1(Input)
  Sum/1 -> Gain/1
  In2/1 -> Sum/2
  Wind_plant1/1 -> Sum/1

== system Wind_Harness/Wind Plant/Detailed/Wind Turbine and Converters/Wind Plant/Back-to-Back Converters/Switching/Grid Side Converter/Pulse Generation1 ==
  G : Inport
  Constant : Constant  Value=5
  Subtract : Sum  Inputs=-+
  G1 : Outport  VectorParamsAs1DForOutWhenUnconnected=off
  G2 : Outport  Port=2  VectorParamsAs1DForOutWhenUnconnected=off
  wires:
  G/1 -> Subtract/1, G1/1
  Constant/1 -> Subtract/2
  Subtract/1 -> G2/1

== system Wind_Harness/Wind Plant/Detailed/Wind Turbine and Converters/Wind Plant/Back-to-Back Converters/Switching/Machine Side Converter/Pulse Generation ==
  G : Inport
  Constant : Constant  Value=5
  Subtract : Sum  Inputs=-+
  G1 : Outport  VectorParamsAs1DForOutWhenUnconnected=off
  G2 : Outport  Port=2  VectorParamsAs1DForOutWhenUnconnected=off
  wires:
  G/1 -> Subtract/1, G1/1
  Constant/1 -> Subtract/2
  Subtract/1 -> G2/1

== system Wind_Harness/Wind Plant/Detailed/Wind Turbine and Converters/Wind Controller/Wind Grid-side Converter Controller/DC voltage controller & current reference/Subsystem1/V_dc_Controller1/PI ==
  Input : Inport
  Discrete-Time Integrator : DiscreteIntegrator  gainval=Ki_dc  SampleTime=Ts  ICPrevOutput=DiscIntNeverNeededParam  ICPrevScaledInput=DiscIntNeverNeededParam
  Gain1 : Gain  Gain=Kp_dc
  Sum1 : Sum  Inputs=|++
  Unit Delay : UnitDelay  SampleTime=Ts  HasFrameUpgradeWarning=on
  Out2 : Outport
  wires:
  Input/1 -> Discrete-Time Integrator/1, Gain1/1
  Gain1/1 -> Unit Delay/1
  Unit Delay/1 -> Sum1/2
  Sum1/1 -> Out2/1
  Discrete-Time Integrator/1 -> Sum1/1
